simulink model "F16A_MissionActivity"  (R2026a)
settings: Solver=VariableStepDiscrete  MaxStep=Inf
settings Model: DataDictionary=F16A_Functional.sldd  Creator=sdarshan  LastModifiedBy=sdarshan

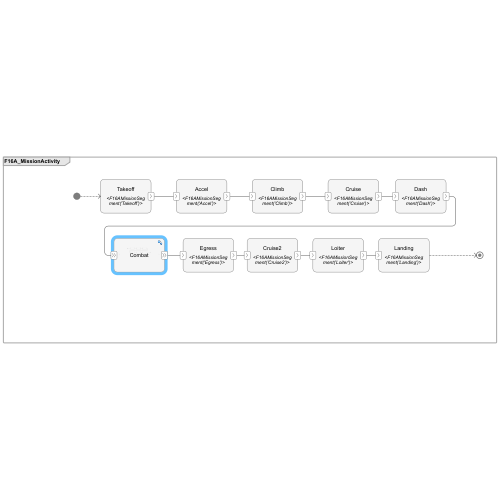
[thumbnail: Simulink's stored preview of the top-level diagram]
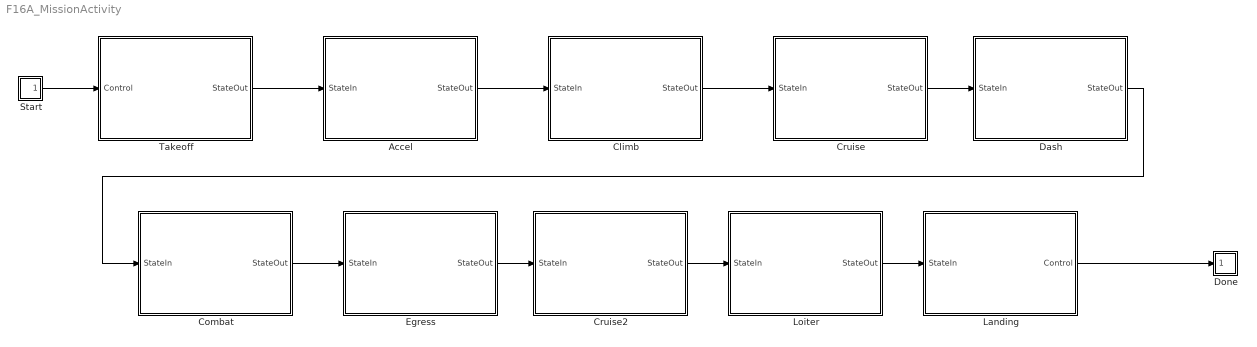
== system F16A_MissionActivity ==
  Accel : Subsystem
      settings: CopyFcn=set_param(gcbh,'LinkStatus','none');
  Climb : Subsystem
      settings: CopyFcn=set_param(gcbh,'LinkStatus','none');
  Combat : Subsystem
      settings: CopyFcn=set_param(gcbh,'LinkStatus','none');
  Cruise : Subsystem
      settings: CopyFcn=set_param(gcbh,'LinkStatus','none');
  Cruise2 : Subsystem
      settings: CopyFcn=set_param(gcbh,'LinkStatus','none');
  Dash : Subsystem
      settings: CopyFcn=set_param(gcbh,'LinkStatus','none');
  Done : Subsystem
      settings: CopyFcn=set_param(gcbh,'LinkStatus','none');
  Egress : Subsystem
      settings: CopyFcn=set_param(gcbh,'LinkStatus','none');
  Landing : Subsystem
      settings: CopyFcn=set_param(gcbh,'LinkStatus','none');
  Loiter : Subsystem
      settings: CopyFcn=set_param(gcbh,'LinkStatus','none');
  Start : Subsystem
      settings: CopyFcn=set_param(gcbh,'LinkStatus','none');
  Takeoff : Subsystem
      settings: CopyFcn=set_param(gcbh,'LinkStatus','none');
  wires:
  Takeoff/1(StateOut) -> Accel/1(StateIn)
  Accel/1(StateOut) -> Climb/1(StateIn)
  Climb/1(StateOut) -> Cruise/1(StateIn)
  Cruise/1(StateOut) -> Dash/1(StateIn)
  Dash/1(StateOut) -> Combat/1(StateIn)
  Combat/1(StateOut) -> Egress/1(StateIn)
  Egress/1(StateOut) -> Cruise2/1(StateIn)
  Cruise2/1(StateOut) -> Loiter/1(StateIn)
  Loiter/1(StateOut) -> Landing/1(StateIn)
  Start/1(Control) -> Takeoff/1(Control)
  Landing/1(Control) -> Done/1(Control)

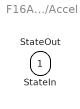
== system F16A_MissionActivity/Accel ==
  StateIn : Inport  OutDataTypeStr=Bus: FlightState
  StateOut : Outport  OutDataTypeStr=Bus: FlightState

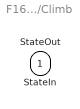
== system F16A_MissionActivity/Climb ==
  StateIn : Inport  OutDataTypeStr=Bus: FlightState
  StateOut : Outport  OutDataTypeStr=Bus: FlightState

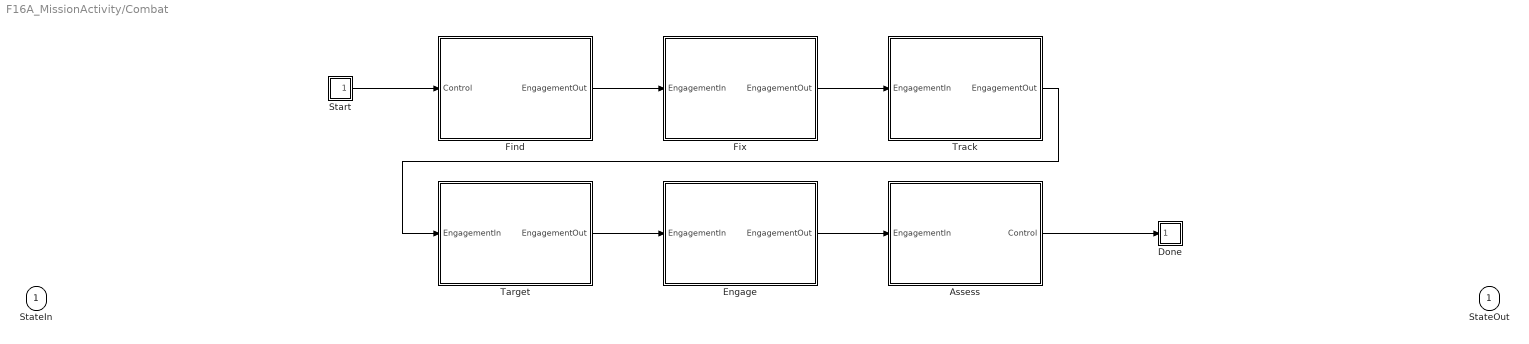
== system F16A_MissionActivity/Combat ==
  StateIn : Inport  OutDataTypeStr=Bus: FlightState
  Assess : Subsystem
      settings: CopyFcn=set_param(gcbh,'LinkStatus','none');
  Done : Subsystem
      settings: CopyFcn=set_param(gcbh,'LinkStatus','none');
  Engage : Subsystem
      settings: CopyFcn=set_param(gcbh,'LinkStatus','none');
  Find : Subsystem
      settings: CopyFcn=set_param(gcbh,'LinkStatus','none');
  Fix : Subsystem
      settings: CopyFcn=set_param(gcbh,'LinkStatus','none');
  Start : Subsystem
      settings: CopyFcn=set_param(gcbh,'LinkStatus','none');
  Target : Subsystem
      settings: CopyFcn=set_param(gcbh,'LinkStatus','none');
  Track : Subsystem
      settings: CopyFcn=set_param(gcbh,'LinkStatus','none');
  StateOut : Outport  OutDataTypeStr=Bus: FlightState
  wires:
  Find/1(EngagementOut) -> Fix/1(EngagementIn)
  Fix/1(EngagementOut) -> Track/1(EngagementIn)
  Track/1(EngagementOut) -> Target/1(EngagementIn)
  Target/1(EngagementOut) -> Engage/1(EngagementIn)
  Engage/1(EngagementOut) -> Assess/1(EngagementIn)
  Start/1(Control) -> Find/1(Control)
  Assess/1(Control) -> Done/1(Control)

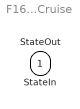
== system F16A_MissionActivity/Cruise ==
  StateIn : Inport  OutDataTypeStr=Bus: FlightState
  StateOut : Outport  OutDataTypeStr=Bus: FlightState

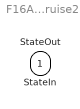
== system F16A_MissionActivity/Cruise2 ==
  StateIn : Inport  OutDataTypeStr=Bus: FlightState
  StateOut : Outport  OutDataTypeStr=Bus: FlightState

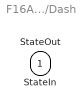
== system F16A_MissionActivity/Dash ==
  StateIn : Inport  OutDataTypeStr=Bus: FlightState
  StateOut : Outport  OutDataTypeStr=Bus: FlightState

== system F16A_MissionActivity/Done ==
  Control : Inport

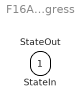
== system F16A_MissionActivity/Egress ==
  StateIn : Inport  OutDataTypeStr=Bus: FlightState
  StateOut : Outport  OutDataTypeStr=Bus: FlightState

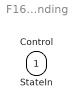
== system F16A_MissionActivity/Landing ==
  StateIn : Inport  OutDataTypeStr=Bus: FlightState
  Control : Outport

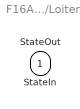
== system F16A_MissionActivity/Loiter ==
  StateIn : Inport  OutDataTypeStr=Bus: FlightState
  StateOut : Outport  OutDataTypeStr=Bus: FlightState

== system F16A_MissionActivity/Start ==
  Control : Outport

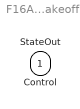
== system F16A_MissionActivity/Takeoff ==
  Control : Inport
  StateOut : Outport  OutDataTypeStr=Bus: FlightState

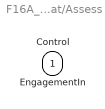
== system F16A_MissionActivity/Combat/Assess ==
  EngagementIn : Inport  OutDataTypeStr=Bus: EngagementData
  Control : Outport

== system F16A_MissionActivity/Combat/Done ==
  Control : Inport

== system F16A_MissionActivity/Combat/Engage ==
  EngagementIn : Inport  OutDataTypeStr=Bus: EngagementData
  EngagementOut : Outport  OutDataTypeStr=Bus: EngagementData

== system F16A_MissionActivity/Combat/Find ==
  Control : Inport
  EngagementOut : Outport  OutDataTypeStr=Bus: EngagementData

== system F16A_MissionActivity/Combat/Fix ==
  EngagementIn : Inport  OutDataTypeStr=Bus: EngagementData
  EngagementOut : Outport  OutDataTypeStr=Bus: EngagementData

== system F16A_MissionActivity/Combat/Start ==
  Control : Outport

== system F16A_MissionActivity/Combat/Target ==
  EngagementIn : Inport  OutDataTypeStr=Bus: EngagementData
  EngagementOut : Outport  OutDataTypeStr=Bus: EngagementData

== system F16A_MissionActivity/Combat/Track ==
  EngagementIn : Inport  OutDataTypeStr=Bus: EngagementData
  EngagementOut : Outport  OutDataTypeStr=Bus: EngagementData
